simulink model "lazo_cerrado"  (R2019a)
settings: Solver=VariableStepAuto  StartTime=0.0  StopTime=10.0  RelTol=1e-3
values from neighbouring files (symbols this model uses):
  den = [34709393649091889, 8873737467196072166715, 24583972753858281030182000, 42460474904292344280000000]    [motor_generador_sim.m]
  K_h = 1.58    [motor_generador_sim.m]
  K_s = 0.003    [motor_generador_sim.m]
  num = [143134928095778949120000, 36192688961361248563200000000]    [motor_generador_sim.m]
  T_h = 0.47    [motor_generador_sim.m]
libraries: simulink x1, simulink_extras x1
settings Model: Creator=lakat  LastModifiedBy=lakat

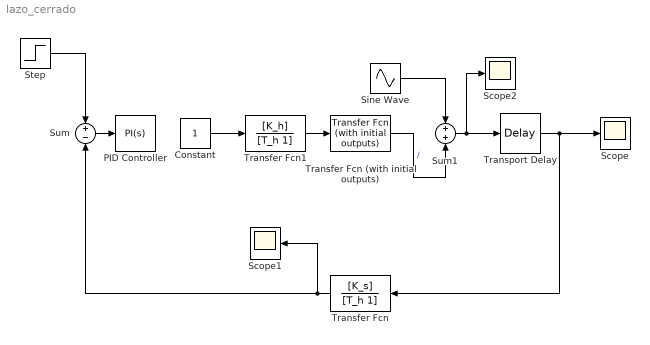
== system lazo_cerrado ==
  Constant : Constant
  PID Controller : simulink/Continuous/PID Controller  Controller=PI  Form=Parallel  TimeDomain=Continuous-time  SampleTime=-1  IntegratorMethod=Forward Euler  FilterMethod=Forward Euler  ControllerParametersSource=internal  P=0.14118615660184  I=0.146559969754698  D=0.185283576593873  UseFilter=on  N=185.830450712222  TunerSelectOption=Transfer Function Based (PID Tuner App)  InitialConditionSource=internal  InitialConditionForIntegrator=0  InitialConditionForFilter=0  DifferentiatorICPrevScaledInput=0  ExternalReset=none  TrackingMode=off  Kt=1  LimitOutput=off  UpperSaturationLimit=inf  LowerSaturationLimit=-inf  LinearizeAsGain=on  AntiWindupMode=none  Kb=1  POutMin=[]  POutMax=[]  IOutMin=[]  IOutMax=[]  DOutMin=[]  DOutMax=[]  NOutMin=[]  NOutMax=0  SumOutMin=[]  SumOutMax=[]  SaturationOutMin=[]  SaturationOutMax=[]  PParamMin=[]  PParamMax=[]  IParamMin=[]  IParamMax=[]  DParamMin=[]  DParamMax=[]  NParamMin=[]  NParamMax=[]  KbParamMin=[]  KbParamMax=[]  KtParamMin=[]  KtParamMax=[]  KbOutMin=[]  KbOutMax=[]  KtOutMin=[]  KtOutMax=[]  IntegratorOutMin=[]  IntegratorOutMax=[]  FilterOutMin=[]  FilterOutMax=[]  SumI1OutMin=[]  SumI1OutMax=[]  SumI2OutMin=[]  SumI2OutMax=[]  SumI3OutMin=[]  SumI3OutMax=[]  SumI4OutMin=[]  SumI4OutMax=[]  SumDOutMin=[]  SumDOutMax=[]  DifferentiatorOutMin=[]  DifferentiatorOutMax=[]  FilterDiffOutCoefMin=[]  FilterDiffOutCoefMax=[]  ReciprocalOutMin=[]  ReciprocalOutMax=[]  SumDenOutMin=[]  SumDenOutMax=[]  SumNumOutMin=[]  SumNumOutMax=[]  DivideOutMin=[]  DivideOutMax=[]  IntegratorContinuousStateAttributes=''  IntegratorStateMustResolveToSignalObject=off  IntegratorRTWStateStorageClass=Auto  FilterContinuousStateAttributes=''  FilterStateMustResolveToSignalObject=off  FilterRTWStateStorageClass=Auto  ParallelPVariant=InternalParameters  IdealPVariant=Disabled  IVariant=InternalParameters  DVariant=Disabled  IntegratorVariant=Continuous  SatVariant=Disabled  AWVariant=Passthrough  PCopyVariant=Disabled  TRVariant=Disabled  FdbkBlocksVariant=Forward  IdealPFdbkVariant=Disabled  SatFdbkVariant=Disabled  DerivativeFilterVariant=Disabled  NVariant=Disabled  NCopyVariant=Disabled_SignalSpec  FilterICVariant=Disabled  IntegratorICVariant=InternalICs  ExternalResetVariant=Disabled  TRSumVariant=Passthrough  SumFdbkVariant=Disabled  SumVariant=Sum_PI
  Scope : Scope
  Scope1 : Scope
  Scope2 : Scope
  Sine Wave : Sin  Frequency=2513  SampleTime=0
  Step : Step  After=1000  SampleTime=0
  Sum : Sum  Inputs=+-
  Sum1 : Sum
  Transfer Fcn : TransferFcn  Description=Sensor  Numerator=[K_s]  Denominator=[T_h 1]  ContinuousStateAttributes='sensor'
  Transfer Fcn (with initial outputs) : simulink_extras/Additional Linear/Transfer Fcn (with initial outputs)  Description=Función de transferencia del sistema, con las condiciones iniciales  N=num  D=den  Y0=1500  U0=2
  Transfer Fcn1 : TransferFcn  Numerator=[K_h]  Denominator=[T_h 1]  ContinuousStateAttributes='convertidor'
  Transport Delay : TransportDelay  DelayTime=0.1
  wires:
  Transfer Fcn1/1 -> Transfer Fcn (with initial outputs)/1
  Step/1 -> Sum/1
  Transfer Fcn/1 -> Scope1/1, Sum/2
  Sum/1 -> PID Controller/1
  Transport Delay/1 -> Transfer Fcn/1, Scope/1
  Sum1/1 -> Scope2/1, Transport Delay/1
  Transfer Fcn (with initial outputs)/1 -> Sum1/2  "/"
  Sine Wave/1 -> Sum1/1
  Constant/1 -> Transfer Fcn1/1
